simulink model "example_4dof_sl"  (R2021a)
settings: Solver=VariableStepAuto  StartTime=0.0  StopTime=100  RelTol=1e-3
values from neighbouring files (symbols this model uses):
  Cf = 0.4*2*(Kf*m2f)^0.5    (= 1923.09929188)    [parameters.m]
  Cr = 0.4*2*(Kr*m2r)^0.5    (= 1980.32142573)    [parameters.m]
  Hp = 0.16    [parameters.m]
  Ip = 2000/2    (= 1000)    [parameters.m]
  Kf = Kfo/Lvf^2    (= 19525.6318975)    [parameters.m]
  Kr = Kro/Lvr^2    (= 23654.1748047)    [parameters.m]
  Kt = 300000    [parameters.m]
  Lf = m2r/m2*wb    (= 1.19956486486)    [parameters.m]
  Lr = m2f/m2*wb    (= 1.37043513514)    [parameters.m]
  m1f = 30    [parameters.m]
  m1r = 30    [parameters.m]
  m2 = m2f + m2r    (= 555)    [parameters.m]
libraries: simulink x1
settings Model: Creator=hmiyagaw  LastModifiedBy=hmiyagaw

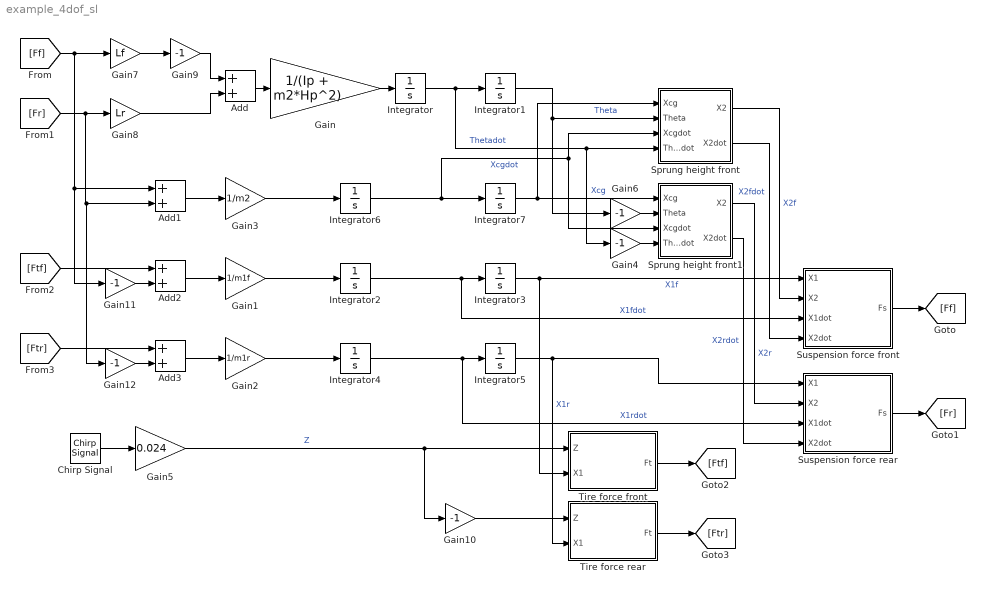
== system example_4dof_sl ==
  Add{,1..3} (4 alike) : Sum
  Chirp Signal : simulink/Sources/Chirp Signal  f1=0  T=100  f2=10
  Gain : Gain  Gain=1/(Ip + m2*Hp^2)
  Gain1 : Gain  Gain=1/m1f
  Gain{4,6,9..12} (6 alike) : Gain  Gain=-1
  Gain2 : Gain  Gain=1/m1r
  Gain3 : Gain  Gain=1/m2
  Gain5 : Gain  Gain=0.024
  Gain7 : Gain  Gain=Lf
  Gain8 : Gain  Gain=Lr
  Integrator{,1..7} (8 alike) : Integrator
  Sprung height front : Subsystem  mask(Sprung Height){L=Lf}
      mask prompts: L "Length from CG[m]"
      mask help: X2 = Xcg - theta*L
  Sprung height front1 : Subsystem  mask(Sprung Height){L=Lr}
      mask prompts: L "Length from CG[m]"
      mask help: X2 = Xcg - theta*L
  Suspension force front : Subsystem  mask(Suspension Force){K=Kf, C=Cf}
      mask prompts: K "Stiffness [N/m]"; C "Dumper [N/(m/s)]"
      mask help: Fs = K(X1-X2) + C(X1dot-X2dot)
  Suspension force rear : Subsystem  mask(Suspension Force){K=Kr, C=Cr}
      mask prompts: K "Stiffness [N/m]"; C "Dumper [N/(m/s)]"
      mask help: Fs = K(X1-X2) + C(X1dot-X2dot)
  Tire force front : Subsystem  mask(Tire Force){K=Kt}
      mask prompts: K "Stiffness [N/m]"
      mask help: Ft = Kt ( Z - X1 )
  Tire force rear : Subsystem  mask(Tire Force){K=Kt}
      mask prompts: K "Stiffness [N/m]"
      mask help: Ft = Kt ( Z - X1 )
  wires:
  Integrator/1 -> Sprung height front/4(Thetadot), Gain4/1, Integrator1/1  "Thetadot"
  Integrator1/1 -> Sprung height front/2(Theta), Gain6/1  "Theta"
  Integrator3/1 -> Tire force front/2(X1), Suspension force front/1(X1)  "X1f"
  Integrator2/1 -> Suspension force front/3(X1dot), Integrator3/1  "X1fdot"
  Integrator4/1 -> Suspension force rear/3(X1dot), Integrator5/1  "X1rdot"
  Integrator5/1 -> Tire force rear/2(X1), Suspension force rear/1(X1)  "X1r"
  Gain/1 -> Integrator/1
  Gain1/1 -> Integrator2/1
  Gain2/1 -> Integrator4/1
  Gain3/1 -> Integrator6/1
  Integrator6/1 -> Sprung height front1/3(Xcgdot), Sprung height front/3(Xcgdot), Integrator7/1  "Xcgdot"
  Integrator7/1 -> Sprung height front1/1(Xcg), Sprung height front/1(Xcg)  "Xcg"
  Chirp Signal/1 -> Gain5/1
  Add/1 -> Gain/1
  Add1/1 -> Gain3/1
  Add2/1 -> Gain1/1
  Add3/1 -> Gain2/1
  Sprung height front/1(X2) -> Suspension force front/2(X2)  "X2f"
  Sprung height front1/1(X2) -> Suspension force rear/2(X2)  "X2r"
  Sprung height front/2(X2dot) -> Suspension force front/4(X2dot)  "X2fdot"
  Sprung height front1/2(X2dot) -> Suspension force rear/4(X2dot)  "X2rdot"
  Suspension force front/1(Fs) -> [Ff]
  Suspension force rear/1(Fs) -> [Fr]
  [Ff] -> Gain7/1, Gain11/1, Add1/1
  [Fr] -> Gain12/1, Add1/2, Gain8/1
  Gain7/1 -> Gain9/1
  Gain5/1 -> Gain10/1, Tire force front/1(Z)  "Z"
  Gain10/1 -> Tire force rear/1(Z)
  Tire force front/1(Ft) -> [Ftf]
  Tire force rear/1(Ft) -> [Ftr]
  [Ftf] -> Add2/1
  [Ftr] -> Add3/1
  Gain11/1 -> Add2/2
  Gain12/1 -> Add3/2
  Gain6/1 -> Sprung height front1/2(Theta)
  Gain4/1 -> Sprung height front1/4(Thetadot)
  Gain8/1 -> Add/2
  Gain9/1 -> Add/1

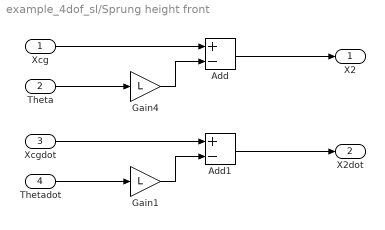
== system example_4dof_sl/Sprung height front ==
  Xcg : Inport
  Theta : Inport  Port=2
  Xcgdot : Inport  Port=3
  Thetadot : Inport  Port=4
  Add : Sum  Inputs=+-
  Add1 : Sum  Inputs=+-
  Gain1 : Gain  Gain=L
  Gain4 : Gain  Gain=L
  X2 : Outport
  X2dot : Outport  Port=2
  wires:
  Xcg/1 -> Add/1
  Gain4/1 -> Add/2
  Theta/1 -> Gain4/1
  Add/1 -> X2/1
  Add1/1 -> X2dot/1
  Gain1/1 -> Add1/2
  Xcgdot/1 -> Add1/1
  Thetadot/1 -> Gain1/1

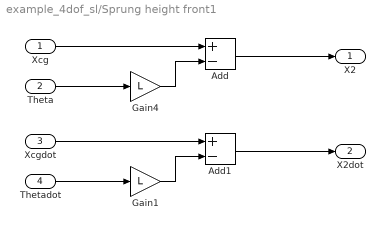
== system example_4dof_sl/Sprung height front1 ==
  Xcg : Inport
  Theta : Inport  Port=2
  Xcgdot : Inport  Port=3
  Thetadot : Inport  Port=4
  Add : Sum  Inputs=+-
  Add1 : Sum  Inputs=+-
  Gain1 : Gain  Gain=L
  Gain4 : Gain  Gain=L
  X2 : Outport
  X2dot : Outport  Port=2
  wires:
  Thetadot/1 -> Gain1/1
  Xcgdot/1 -> Add1/1
  Gain1/1 -> Add1/2
  Add1/1 -> X2dot/1
  Add/1 -> X2/1
  Theta/1 -> Gain4/1
  Gain4/1 -> Add/2
  Xcg/1 -> Add/1

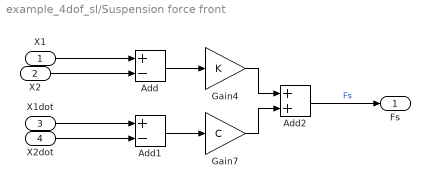
== system example_4dof_sl/Suspension force front ==
  X1 : Inport
  X2 : Inport  Port=2
  X1dot : Inport  Port=3
  X2dot : Inport  Port=4
  Add : Sum  Inputs=+-
  Add1 : Sum  Inputs=+-
  Add2 : Sum
  Gain4 : Gain  Gain=K
  Gain7 : Gain  Gain=C
  Fs : Outport
  wires:
  Add2/1 -> Fs/1  "Fs"
  X2/1 -> Add/2
  Add1/1 -> Gain7/1
  Gain7/1 -> Add2/2
  Gain4/1 -> Add2/1
  X1/1 -> Add/1
  X1dot/1 -> Add1/1
  X2dot/1 -> Add1/2
  Add/1 -> Gain4/1

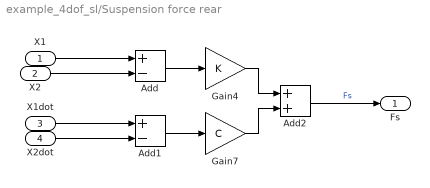
== system example_4dof_sl/Suspension force rear ==
  X1 : Inport
  X2 : Inport  Port=2
  X1dot : Inport  Port=3
  X2dot : Inport  Port=4
  Add : Sum  Inputs=+-
  Add1 : Sum  Inputs=+-
  Add2 : Sum
  Gain4 : Gain  Gain=K
  Gain7 : Gain  Gain=C
  Fs : Outport
  wires:
  Add/1 -> Gain4/1
  X2dot/1 -> Add1/2
  X1dot/1 -> Add1/1
  X1/1 -> Add/1
  Gain4/1 -> Add2/1
  Gain7/1 -> Add2/2
  Add1/1 -> Gain7/1
  X2/1 -> Add/2
  Add2/1 -> Fs/1  "Fs"

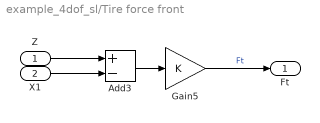
== system example_4dof_sl/Tire force front ==
  Z : Inport
  X1 : Inport  Port=2
  Add3 : Sum  Inputs=+-
  Gain5 : Gain  Gain=K
  Ft : Outport
  wires:
  Gain5/1 -> Ft/1  "Ft"
  Z/1 -> Add3/1
  Add3/1 -> Gain5/1
  X1/1 -> Add3/2

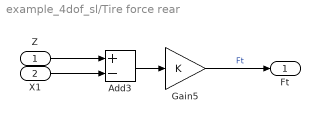
== system example_4dof_sl/Tire force rear ==
  Z : Inport
  X1 : Inport  Port=2
  Add3 : Sum  Inputs=+-
  Gain5 : Gain  Gain=K
  Ft : Outport
  wires:
  X1/1 -> Add3/2
  Add3/1 -> Gain5/1
  Z/1 -> Add3/1
  Gain5/1 -> Ft/1  "Ft"
